simulink model "experiment4_anto_conctrol"  (R2022a)
settings: Solver=VariableStepAuto  StartTime=0.0  StopTime=100  RelTol=1e-3
settings Model: Creator=slack  LastModifiedBy=slack

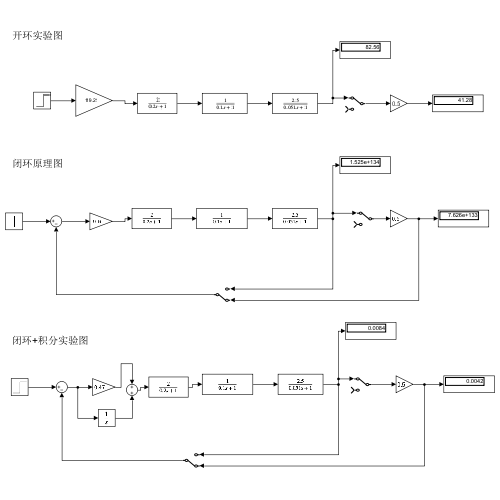
[thumbnail: Simulink's stored preview of the top-level diagram]
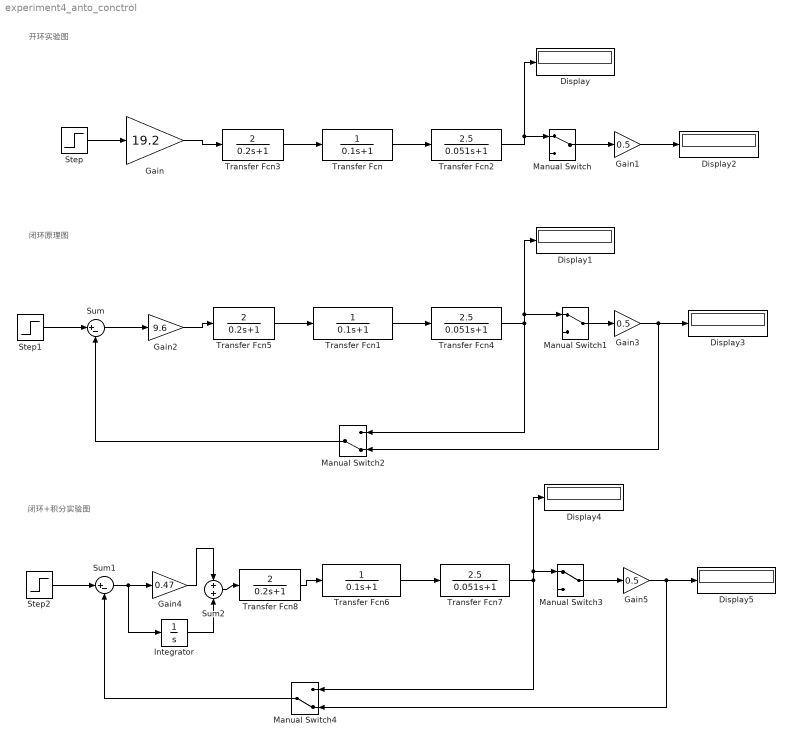
== system experiment4_anto_conctrol ==
  note: 开环实验图
  note: 闭环原理图
  note: 闭环+积分实验图
  Display{,1..5} (6 alike) : Display
  Gain : Gain  Gain=19.2
  Gain1 : Gain  Gain=0.5
  Gain2 : Gain  Gain=9.6
  Gain3 : Gain  Gain=0.5
  Gain4 : Gain  Gain=0.47
  Gain5 : Gain  Gain=0.5
  Integrator : Integrator
  Manual Switch : ManualSwitch
  Manual Switch1 : ManualSwitch
  Manual Switch2 : ManualSwitch  CurrentSetting=0
  Manual Switch3 : ManualSwitch
  Manual Switch4 : ManualSwitch  CurrentSetting=0
  Step : Step  After=0.86  SampleTime=0
  Step1 : Step  After=0.86  SampleTime=0
  Step2 : Step  After=0.0042  SampleTime=0
  Sum : Sum  Inputs=|+-
  Sum1 : Sum  Inputs=|+-
  Sum2 : Sum
  Transfer Fcn : TransferFcn  Denominator=[0.1 1]
  Transfer Fcn1 : TransferFcn  Denominator=[0.1 1]
  Transfer Fcn2 : TransferFcn  Numerator=[2.5]  Denominator=[0.051 1]
  Transfer Fcn3 : TransferFcn  Numerator=[2]  Denominator=[0.2 1]
  Transfer Fcn4 : TransferFcn  Numerator=[2.5]  Denominator=[0.051 1]
  Transfer Fcn5 : TransferFcn  Numerator=[2]  Denominator=[0.2 1]
  Transfer Fcn6 : TransferFcn  Denominator=[0.1 1]
  Transfer Fcn7 : TransferFcn  Numerator=[2.5]  Denominator=[0.051 1]
  Transfer Fcn8 : TransferFcn  Numerator=[2]  Denominator=[0.2 1]
  wires:
  Step/1 -> Gain/1
  Gain/1 -> Transfer Fcn3/1
  Transfer Fcn3/1 -> Transfer Fcn/1
  Transfer Fcn/1 -> Transfer Fcn2/1
  Transfer Fcn2/1 -> Display/1, Manual Switch/1
  Manual Switch/1 -> Gain1/1
  Gain1/1 -> Display2/1
  Manual Switch1/1 -> Gain3/1
  Transfer Fcn4/1 -> Manual Switch2/1, Display1/1, Manual Switch1/1
  Transfer Fcn1/1 -> Transfer Fcn4/1
  Gain3/1 -> Display3/1, Manual Switch2/2
  Transfer Fcn5/1 -> Transfer Fcn1/1
  Gain2/1 -> Transfer Fcn5/1
  Step1/1 -> Sum/1
  Sum/1 -> Gain2/1
  Manual Switch2/1 -> Sum/2
  Gain5/1 -> Display5/1, Manual Switch4/2
  Transfer Fcn6/1 -> Transfer Fcn7/1
  Manual Switch3/1 -> Gain5/1
  Transfer Fcn7/1 -> Manual Switch4/1, Display4/1, Manual Switch3/1
  Transfer Fcn8/1 -> Transfer Fcn6/1
  Manual Switch4/1 -> Sum1/2
  Step2/1 -> Sum1/1
  Sum1/1 -> Integrator/1, Gain4/1
  Gain4/1 -> Sum2/1
  Sum2/1 -> Transfer Fcn8/1
  Integrator/1 -> Sum2/2
